simulink model "MFinal"  (R2024b)
settings: configuration reference "STM32H7_Config" (kept outside this file)
settings Model: DataDictionary=Master_Dictionary.sldd  EnableAccessToBaseWorkspace=off  Creator=torni  LastModifiedBy=William
settings ConfigSetRef: SourceName=STM32H7_Config

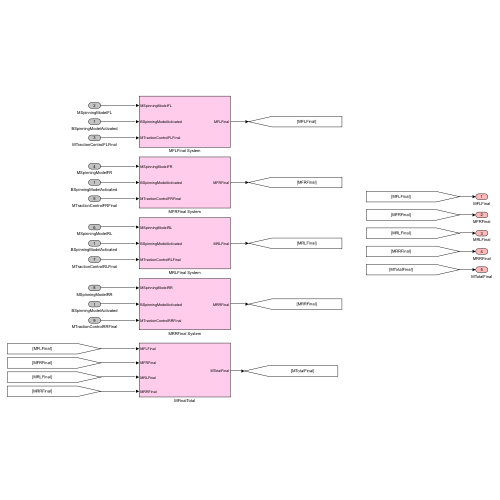
[thumbnail: Simulink's stored preview of the top-level diagram]
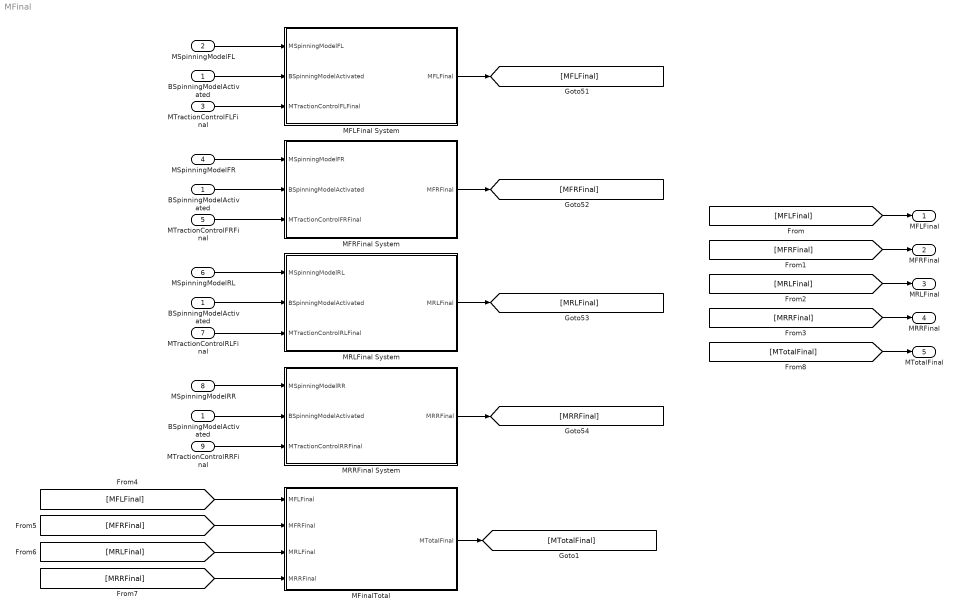
== system MFinal ==
  BSpinningModelActivated : Inport  OutDataTypeStr=boolean
  MSpinningModelFL : Inport  Port=2  OutDataTypeStr=double
  "MTractionControlFLFinal " : Inport  Port=3  OutDataTypeStr=double
  MSpinningModelFR : Inport  Port=4  OutDataTypeStr=double
  "MTractionControlFRFinal " : Inport  Port=5  OutDataTypeStr=double
  MSpinningModelRL : Inport  Port=6  OutDataTypeStr=double
  MTractionControlRLFinal : Inport  Port=7  OutDataTypeStr=double
  MSpinningModelRR : Inport  Port=8  OutDataTypeStr=double
  "MTractionControlRRFinal " : Inport  Port=9  OutDataTypeStr=double
  "BSpinningModelActivated " : InportShadow  OutDataTypeStr=boolean
  "BSpinningModelActivated " : InportShadow  OutDataTypeStr=boolean
  "BSpinningModelActivated " : InportShadow  OutDataTypeStr=boolean
  MFLFinal System : Subsystem
  MFRFinal System : Subsystem
  MFinalTotal : Subsystem
  MRLFinal System : Subsystem
  MRRFinal System : Subsystem
  MFLFinal : Outport  OutDataTypeStr=double  VectorParamsAs1DForOutWhenUnconnected=off
  MFRFinal : Outport  Port=2  OutDataTypeStr=double  VectorParamsAs1DForOutWhenUnconnected=off
  MRLFinal : Outport  Port=3  OutDataTypeStr=double  VectorParamsAs1DForOutWhenUnconnected=off
  MRRFinal : Outport  Port=4  OutDataTypeStr=double  VectorParamsAs1DForOutWhenUnconnected=off
  MTotalFinal : Outport  Port=5  OutDataTypeStr=double  VectorParamsAs1DForOutWhenUnconnected=off
  wires:
  MSpinningModelFL/1 -> MFLFinal System/1(MSpinningModelFL)
  BSpinningModelActivated/1 -> MFLFinal System/2(BSpinningModelActivated)
  "MTractionControlFLFinal "/1 -> MFLFinal System/3("MTractionControlFLFinal ")
  MSpinningModelFR/1 -> MFRFinal System/1(MSpinningModelFR)
  "BSpinningModelActivated "/1 -> MFRFinal System/2(BSpinningModelActivated)
  "MTractionControlFRFinal "/1 -> MFRFinal System/3("MTractionControlFRFinal ")
  MSpinningModelRL/1 -> MRLFinal System/1(MSpinningModelRL)
  MTractionControlRLFinal/1 -> MRLFinal System/3(MTractionControlRLFinal)
  "BSpinningModelActivated "/1 -> MRLFinal System/2(BSpinningModelActivated)
  "BSpinningModelActivated "/1 -> MRRFinal System/2(BSpinningModelActivated)
  MSpinningModelRR/1 -> MRRFinal System/1(MSpinningModelRR)
  "MTractionControlRRFinal "/1 -> MRRFinal System/3("MTractionControlRRFinal ")
  MFLFinal System/1(MFLFinal) -> [MFLFinal]
  MFRFinal System/1(MFRFinal) -> [MFRFinal]
  MRRFinal System/1(MRRFinal) -> [MRRFinal]
  MRLFinal System/1(MRLFinal) -> [MRLFinal]
  [MFLFinal] -> MFLFinal/1
  [MFRFinal] -> MFRFinal/1
  [MRLFinal] -> MRLFinal/1
  [MRRFinal] -> MRRFinal/1
  [MFLFinal] -> MFinalTotal/1(MFLFinal)
  [MFRFinal] -> MFinalTotal/2(MFRFinal)
  [MRLFinal] -> MFinalTotal/3(MRLFinal)
  [MRRFinal] -> MFinalTotal/4(MRRFinal)
  MFinalTotal/1(MTotalFinal) -> [MTotalFinal]
  [MTotalFinal] -> MTotalFinal/1

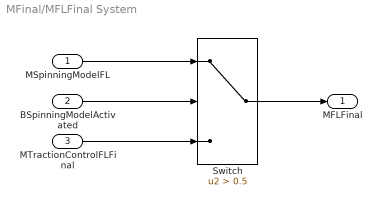
== system MFinal/MFLFinal System ==
  MSpinningModelFL : Inport  OutDataTypeStr=double
  BSpinningModelActivated : Inport  Port=2  OutDataTypeStr=boolean
  "MTractionControlFLFinal " : Inport  Port=3  OutDataTypeStr=double
  Switch : Switch  Criteria=u2 > Threshold  Threshold=0.5  SaturateOnIntegerOverflow=off  InputSameDT=off
  MFLFinal : Outport  OutDataTypeStr=double  VectorParamsAs1DForOutWhenUnconnected=off
  wires:
  BSpinningModelActivated/1 -> Switch/2
  MSpinningModelFL/1 -> Switch/1
  Switch/1 -> MFLFinal/1
  "MTractionControlFLFinal "/1 -> Switch/3

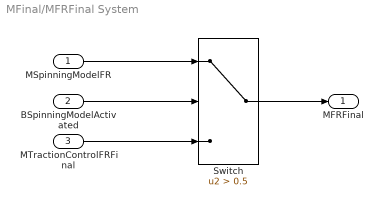
== system MFinal/MFRFinal System ==
  MSpinningModelFR : Inport  OutDataTypeStr=double
  BSpinningModelActivated : Inport  Port=2  OutDataTypeStr=boolean
  "MTractionControlFRFinal " : Inport  Port=3  OutDataTypeStr=double
  Switch : Switch  Criteria=u2 > Threshold  Threshold=0.5  SaturateOnIntegerOverflow=off  InputSameDT=off
  MFRFinal : Outport  OutDataTypeStr=double  VectorParamsAs1DForOutWhenUnconnected=off
  wires:
  "MTractionControlFRFinal "/1 -> Switch/3
  Switch/1 -> MFRFinal/1
  MSpinningModelFR/1 -> Switch/1
  BSpinningModelActivated/1 -> Switch/2

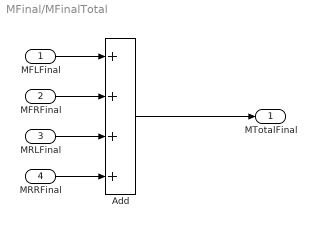
== system MFinal/MFinalTotal ==
  MFLFinal : Inport  OutDataTypeStr=double
  MFRFinal : Inport  Port=2  OutDataTypeStr=double
  MRLFinal : Inport  Port=3  OutDataTypeStr=double
  MRRFinal : Inport  Port=4  OutDataTypeStr=double
  Add : Sum  Inputs=++++
  MTotalFinal : Outport  VectorParamsAs1DForOutWhenUnconnected=off
  wires:
  MFLFinal/1 -> Add/1
  MFRFinal/1 -> Add/2
  MRLFinal/1 -> Add/3
  MRRFinal/1 -> Add/4
  Add/1 -> MTotalFinal/1

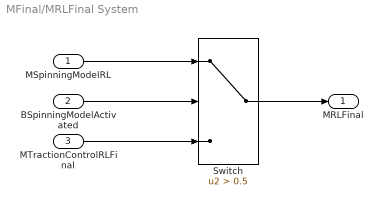
== system MFinal/MRLFinal System ==
  MSpinningModelRL : Inport  OutDataTypeStr=double
  BSpinningModelActivated : Inport  Port=2  OutDataTypeStr=boolean
  MTractionControlRLFinal : Inport  Port=3  OutDataTypeStr=double
  Switch : Switch  Criteria=u2 > Threshold  Threshold=0.5  SaturateOnIntegerOverflow=off  InputSameDT=off
  MRLFinal : Outport  OutDataTypeStr=double  VectorParamsAs1DForOutWhenUnconnected=off
  wires:
  BSpinningModelActivated/1 -> Switch/2
  MSpinningModelRL/1 -> Switch/1
  Switch/1 -> MRLFinal/1
  MTractionControlRLFinal/1 -> Switch/3

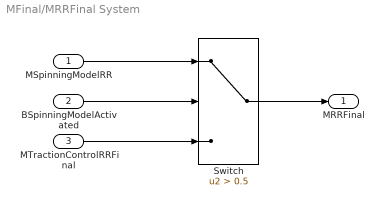
== system MFinal/MRRFinal System ==
  MSpinningModelRR : Inport  OutDataTypeStr=double
  BSpinningModelActivated : Inport  Port=2  OutDataTypeStr=boolean
  "MTractionControlRRFinal " : Inport  Port=3  OutDataTypeStr=double
  Switch : Switch  Criteria=u2 > Threshold  Threshold=0.5  SaturateOnIntegerOverflow=off  InputSameDT=off
  MRRFinal : Outport  OutDataTypeStr=double  VectorParamsAs1DForOutWhenUnconnected=off
  wires:
  "MTractionControlRRFinal "/1 -> Switch/3
  Switch/1 -> MRRFinal/1
  MSpinningModelRR/1 -> Switch/1
  BSpinningModelActivated/1 -> Switch/2
